simulink model "testEncoderRead"  (R2018b)
settings: Solver=FixedStepDiscrete  StartTime=0.0  StopTime=10.0  FixedStep=.1  RelTol=1e-3  EnableMultiTasking=on
libraries: arduinolib x5
settings Model: ExtModeTrigDuration=2  Creator=KSURCT General  LastModifiedBy=KSURCT Officers
settings OptimizationCC: EnhancedBackFolding=on  PassReuseOutputArgsAs=Individual arguments  MaxStackSize=64  OptimizeBlockOrder=speed  DifferentSizesBufferReuse=on  OptimizationCustomize=off
settings DebuggingCC: ParameterTunabilityLossMsg=error
settings HardwareCC: ProdBitPerPointer=32  ProdBitPerSizeT=32  ProdBitPerPtrDiffT=32  ProdLargestAtomicInteger=Long  ProdLargestAtomicFloat=Double  ProdWordSize=32  ProdHWDeviceType=ARM Compatible->ARM Cortex
settings SFSimCC: MATLABDynamicMemAlloc=off
settings RTWCC: SystemTargetFile=ert.tlc  HardwareBoard=Arduino Due  TemplateMakefile=ert_default_tmf  GenerateReport=on  Toolchain=Arduino ARM  BuildConfiguration=Faster Runs  IncludeHyperlinkInReport=on  LaunchReport=on  GenerateTraceInfo=on  GenerateTraceReport=on  GenerateTraceReportSl=on  GenerateTraceReportSf=on  GenerateTraceReportEml=on
settings CodeAppCC: ForceParamTrailComments=on  IgnoreCustomStorageClasses=off  OperatorAnnotations=on  SimulinkDataObjDesc=on  SFDataObjDesc=on  InsertBlockDesc=on
settings ERTTargetCC: SupportContinuousTime=on  SupportVariableSizeSignals=on

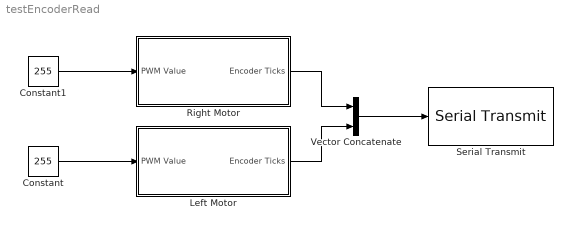
== system testEncoderRead ==
  Constant : Constant  Value=255
  Constant1 : Constant  Value=255
  Left Motor : Subsystem
  Right Motor : Subsystem
  Serial Transmit : arduinolib/Serial Transmit  portNumber=0  sendmode=println  label=right >>  sendformat=Decimal  floatprecision=2  blockPlatform=arduino
      settings: SourceProductName=Simulink Support Package for Arduino Hardware
  Vector Concatenate : Concatenate
  wires:
  Vector Concatenate/1 -> Serial Transmit/1
  Right Motor/1(Encoder Ticks) -> Vector Concatenate/1
  Left Motor/1(Encoder Ticks) -> Vector Concatenate/2
  Constant/1 -> Left Motor/1(PWM Value)
  Constant1/1 -> Right Motor/1(PWM Value)

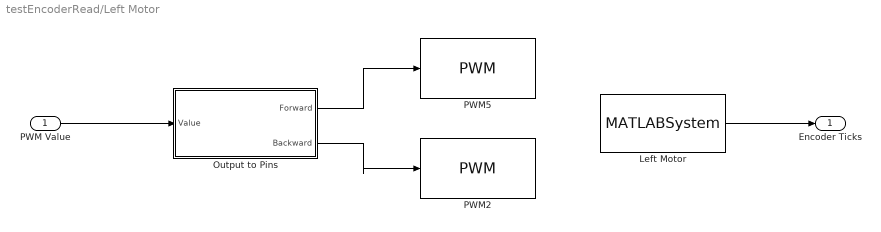
== system testEncoderRead/Left Motor ==
  PWM Value : Inport
  Left Motor : MATLABSystem  System=EncoderRead  pinA=int8(11)  pinB=int8(10)  id=int8(0)  SampleTime=-1
      mask Type: EncoderRead
      mask Display:
      | disp('Source');
      | port_label('output',1,'ticks');
  Output to Pins : Subsystem
  PWM2 : arduinolib/PWM  pinNumber=2  EnableInputFrequency=off  InitialFrequency=2000  InitialDutyCycle=0  NotificationType=None  blockPlatform=arduino
  PWM5 : arduinolib/PWM  pinNumber=3  EnableInputFrequency=off  InitialFrequency=2000  InitialDutyCycle=0  NotificationType=None  blockPlatform=arduino
  Encoder Ticks : Outport
  wires:
  Output to Pins/2("Backward ") -> PWM2/1
  Output to Pins/1(Forward) -> PWM5/1
  PWM Value/1 -> Output to Pins/1(Value)
  Left Motor/1 -> Encoder Ticks/1

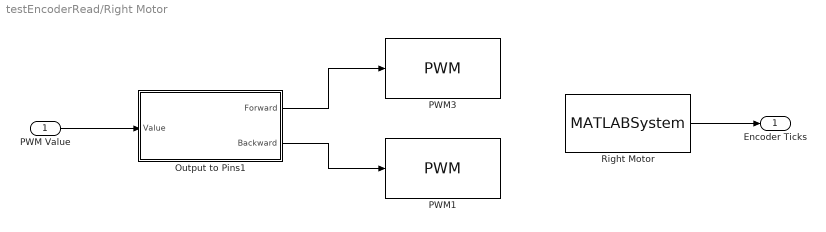
== system testEncoderRead/Right Motor ==
  PWM Value : Inport
  Output to Pins1 : Subsystem
  PWM1 : arduinolib/PWM  pinNumber=4  EnableInputFrequency=off  InitialFrequency=2000  InitialDutyCycle=0  NotificationType=None  blockPlatform=arduino
  PWM3 : arduinolib/PWM  pinNumber=5  EnableInputFrequency=off  InitialFrequency=2000  InitialDutyCycle=0  NotificationType=None  blockPlatform=arduino
  Right Motor : MATLABSystem  System=EncoderRead  pinA=int8(13)  pinB=int8(12)  id=int8(1)  SampleTime=-1
      mask Type: EncoderRead
      mask Display:
      | disp('Source');
      | port_label('output',1,'ticks');
  Encoder Ticks : Outport
  wires:
  Output to Pins1/2("Backward ") -> PWM1/1
  PWM Value/1 -> Output to Pins1/1(Value)
  Output to Pins1/1(Forward) -> PWM3/1
  Right Motor/1 -> Encoder Ticks/1

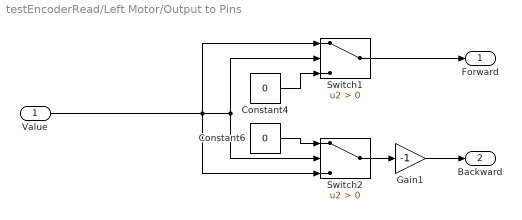
== system testEncoderRead/Left Motor/Output to Pins ==
  Value : Inport
  Constant4 : Constant  Value=0
  Constant6 : Constant  Value=0
  Gain1 : Gain  Gain=-1
  Switch1 : Switch  Criteria=u2 > Threshold
  Switch2 : Switch  Criteria=u2 > Threshold
  Forward : Outport
  "Backward " : Outport  Port=2
  wires:
  Value/1 -> Switch2/2, Switch1/2, Switch2/3, Switch1/1
  Constant4/1 -> Switch1/3
  Gain1/1 -> "Backward "/1
  Switch2/1 -> Gain1/1
  Constant6/1 -> Switch2/1
  Switch1/1 -> Forward/1

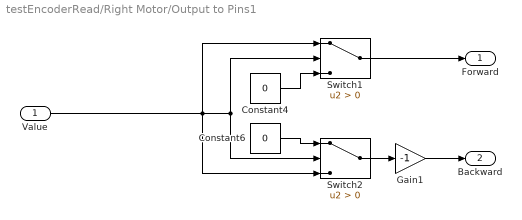
== system testEncoderRead/Right Motor/Output to Pins1 ==
  Value : Inport
  Constant4 : Constant  Value=0
  Constant6 : Constant  Value=0
  Gain1 : Gain  Gain=-1
  Switch1 : Switch  Criteria=u2 > Threshold
  Switch2 : Switch  Criteria=u2 > Threshold
  Forward : Outport
  "Backward " : Outport  Port=2
  wires:
  Switch1/1 -> Forward/1
  Constant6/1 -> Switch2/1
  Switch2/1 -> Gain1/1
  Gain1/1 -> "Backward "/1
  Constant4/1 -> Switch1/3
  Value/1 -> Switch1/1, Switch2/3, Switch1/2, Switch2/2
